simulink model "final_obc1"  (R2022a)
settings: Solver=VariableStepAuto  StartTime=0.0  StopTime=0.7  RelTol=1e-3
values from neighbouring files (symbols this model uses):
  ccControl_Kaw = 0    [final.mat]
  cvControl_Kaw = 1    [final.mat]
  Ki = 46    [final.mat]
  Kp = 0.22    [final.mat]
  Ts = 5e-06    [final.mat]
  Tsc = 0.0001    [final.mat]
libraries: fl_lib x20, nesl_utility x19, ee_lib x12, eeGeneralControl x6, slpidlib x4, spsPWMGeneratorDCDCLib x4, spsTHDLib x4, eeDcDcVoltageController x1, eePwmGenerator x1
(part 2 of 2)

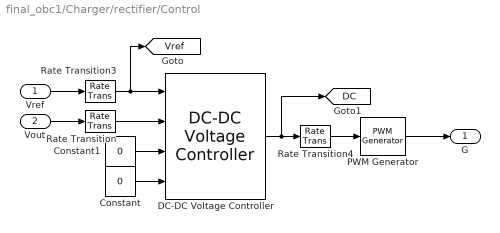
== system final_obc1/Charger/rectifier/Control ==
  Vref : Inport
  Vout : Inport  Port=2
  Constant : Constant  Value=0
  Constant1 : Constant  Value=0
  DC-DC Voltage Controller : eeDcDcVoltageController/DC-DC Voltage Controller  Kp=Kp  Ki=Ki  Kaw=1  up=0.95  lo=0  Ts=Tsc  Tf=0.001  ActVdcFilter=off
      settings: SourceProductBaseCode=PS
  PWM Generator : eePwmGenerator/PWM Generator  CarrCount=Up  Tper=1e-4  Tdelay=0  Ts=Ts
  Rate Transition : RateTransition  OutPortSampleTime=Tsc
  Rate Transition3 : RateTransition  OutPortSampleTime=Tsc
  Rate Transition4 : RateTransition  OutPortSampleTime=Ts
  G : Outport  VectorParamsAs1DForOutWhenUnconnected=off
  tag scope: DC=global, Vref=global
  wires:
  Vref/1 -> Rate Transition3/1
  Rate Transition3/1 -> [Vref], DC-DC Voltage Controller/1
  Vout/1 -> Rate Transition/1
  PWM Generator/1 -> G/1
  DC-DC Voltage Controller/1 -> Rate Transition4/1, [DC]
  Rate Transition4/1 -> PWM Generator/1
  Constant1/1 -> DC-DC Voltage Controller/3
  Constant/1 -> DC-DC Voltage Controller/4
  Rate Transition/1 -> DC-DC Voltage Controller/2

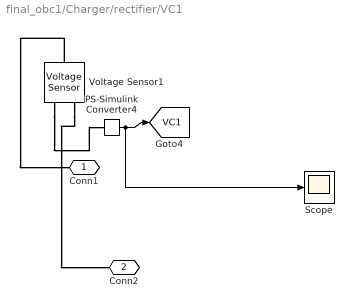
== system final_obc1/Charger/rectifier/VC1 ==
  PS-Simulink Converter4 : nesl_utility/PS-Simulink Converter  PhysicalDomain=network_engine_domain  SubClassName=ps_output  LeftPortType=input  RightPortType=output  PseudoPeriodic=off  Frequencies=[]  VectorFormat=inherit  Unit=inherit  AffineConversion=off
      settings: SourceProductBaseCode=SS,PW,VE
  Scope : Scope
  Voltage Sensor1 : fl_lib/Electrical/Electrical Sensors/Voltage Sensor
      settings: SourceProductBaseCode=PW,SS,VE
  Conn1 : PMIOPort  Side=Left
  Conn2 : PMIOPort  Port=2  Side=Right
  tag scope: VC1=global
  wires:
  PS-Simulink Converter4/1 -> Scope/1, [VC1]
  connections:
  Voltage Sensor1/RConn1 -- PS-Simulink Converter4/LConn1
  Voltage Sensor1/RConn2 -- Conn2/RConn1
  Voltage Sensor1/LConn1 -- Conn1/RConn1

== system final_obc1/Charger/rectifier/VC2 ==
  PS-Simulink Converter5 : nesl_utility/PS-Simulink Converter  PhysicalDomain=network_engine_domain  SubClassName=ps_output  LeftPortType=input  RightPortType=output  PseudoPeriodic=off  Frequencies=[]  VectorFormat=inherit  Unit=inherit  AffineConversion=off
      settings: SourceProductBaseCode=SS,PW,VE
  Voltage Sensor2 : fl_lib/Electrical/Electrical Sensors/Voltage Sensor
      settings: SourceProductBaseCode=PW,SS,VE
  Conn1 : PMIOPort  Side=Left
  Conn2 : PMIOPort  Port=2  Side=Right
  tag scope: VC2=global
  wires:
  PS-Simulink Converter5/1 -> [VC2]
  connections:
  Voltage Sensor2/RConn1 -- PS-Simulink Converter5/LConn1
  Voltage Sensor2/LConn1 -- Conn1/RConn1
  Voltage Sensor2/RConn2 -- Conn2/RConn1

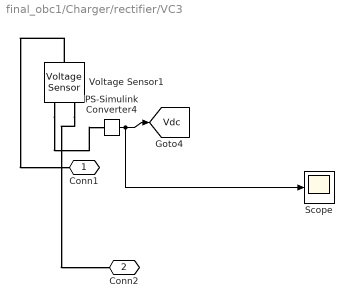
== system final_obc1/Charger/rectifier/VC3 ==
  PS-Simulink Converter4 : nesl_utility/PS-Simulink Converter  PhysicalDomain=network_engine_domain  SubClassName=ps_output  LeftPortType=input  RightPortType=output  PseudoPeriodic=off  Frequencies=[]  VectorFormat=inherit  Unit=inherit  AffineConversion=off
      settings: SourceProductBaseCode=SS,PW,VE
  Scope : Scope
  Voltage Sensor1 : fl_lib/Electrical/Electrical Sensors/Voltage Sensor
      settings: SourceProductBaseCode=PW,SS,VE
  Conn1 : PMIOPort  Side=Left
  Conn2 : PMIOPort  Port=2  Side=Right
  tag scope: Vdc=global
  wires:
  PS-Simulink Converter4/1 -> Scope/1, [Vdc]
  connections:
  Voltage Sensor1/RConn1 -- PS-Simulink Converter4/LConn1
  Voltage Sensor1/RConn2 -- Conn2/RConn1
  Voltage Sensor1/LConn1 -- Conn1/RConn1

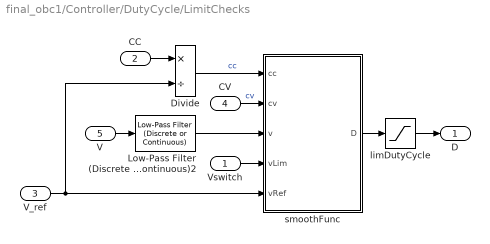
== system final_obc1/Controller/DutyCycle/LimitChecks ==
  Vswitch : Inport
  CC : Inport  Port=2
  V_ref : Inport  Port=3
  CV : Inport  Port=4
  V : Inport  Port=5
  Divide : Product  Inputs=*/
  Low-Pass Filter (Discrete or Continuous)2 : eeGeneralControl/Low-Pass Filter (Discrete or Continuous)  K=1  T=1  B=inf  A=-inf  init_option=Inherited from block input  x0=0  Ts=0
  limDutyCycle : Saturate  UpperLimit=.99  LowerLimit=0.0001
  smoothFunc : MATLAB Function  TreatAsAtomicUnit=on
  D : Outport
  wires:
  V_ref/1 -> Divide/2, smoothFunc/5(vRef)
  CC/1 -> Divide/1
  limDutyCycle/1 -> D/1
  smoothFunc/1(D) -> limDutyCycle/1
  Divide/1 -> smoothFunc/1(cc)  "cc"
  V/1 -> Low-Pass Filter (Discrete or Continuous)2/1
  Vswitch/1 -> smoothFunc/4(vLim)
  CV/1 -> smoothFunc/2(cv)  "cv"
  Low-Pass Filter (Discrete or Continuous)2/1 -> smoothFunc/3(v)

== system final_obc1/Controller/Feedback/SOCcheck ==
  SOC : Inport
  Constant3 : Constant  Value=0.9999
  Constant4 : Constant  Value=0
  MinMax : MinMax  Function=max  Inputs=2
  Subtract : Sum  Inputs=+-
  state : Outport
  wires:
  Constant4/1 -> MinMax/2
  Subtract/1 -> MinMax/1
  Constant3/1 -> Subtract/2
  MinMax/1 -> state/1
  SOC/1 -> Subtract/1

== matlab function final_obc1/Controller/DutyCycle/LimitChecks/smoothFunc ==
  data: cc input; D output; cv input; v input; vLim input; vRef input
function D = Dsmooth(cc,cv,v,vLim,vRef)
    f=min(1,max(0,(v-vLim)/(vRef-vLim)));
    %f=max(1,max(0,(v-vLim)/(vRef-vLim)));
    D=cc*(1-f)+cv*f;
end
